simulink model "TVC_model_simulink"  (R2020b)
settings: Solver=VariableStepAuto  StartTime=0.0  StopTime=60  RelTol=1e-3
values from neighbouring files (symbols this model uses):
  C = [1 0 0 0 0 0 ... (first row only)    [TVC_model.m]
  dt = 0.01    [TVC_model.m]
  g = 9.8    [TVC_model.m]
  I = 0.002    [TVC_model.m]
  K = place(A,B,P)    [TVC_model.m]
  L = 0.1    [TVC_model.m]
  m = 1    [TVC_model.m]
undefined symbols (not defined in the file or in its folder): sigbuilder_block
libraries: simulink x1
settings Model: Creator=govindchari  LastModifiedBy=govindchari

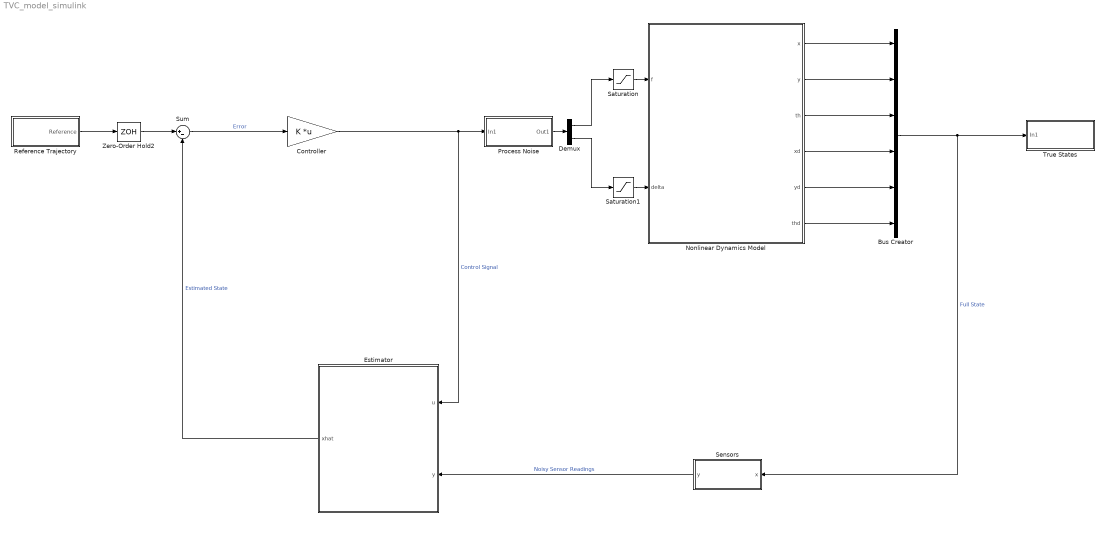
== system TVC_model_simulink ==
  Bus Creator : BusCreator  Inputs=6
  Controller : Gain  Gain=K  Multiplication=Matrix(K*u) (u vector)
  Demux : Demux  Outputs=2
  Estimator : Subsystem
  Nonlinear Dynamics Model : Subsystem
  Process Noise : Subsystem
  Reference Trajectory : Subsystem
  Saturation : Saturate  UpperLimit=m*g  LowerLimit=-m*g
  Saturation1 : Saturate  UpperLimit=0.2  LowerLimit=-0.2
  Sensors : Subsystem
  Sum : Sum  Inputs=|+-
  True States : Subsystem
  Zero-Order Hold2 : ZeroOrderHold  SampleTime=0.01
  wires:
  Nonlinear Dynamics Model/1(x) -> Bus Creator/1
  Nonlinear Dynamics Model/2(y) -> Bus Creator/2
  Nonlinear Dynamics Model/3(th) -> Bus Creator/3
  Nonlinear Dynamics Model/4(xd) -> Bus Creator/4
  Nonlinear Dynamics Model/5(yd) -> Bus Creator/5
  Nonlinear Dynamics Model/6(thd) -> Bus Creator/6
  Bus Creator/1 -> Sensors/1(x), True States/1(In1)  "Full State"
  Demux/1 -> Saturation/1
  Demux/2 -> Saturation1/1
  Sum/1 -> Controller/1  "Error"
  Saturation1/1 -> Nonlinear Dynamics Model/2(delta)
  Saturation/1 -> Nonlinear Dynamics Model/1(f)
  Reference Trajectory/1(Reference) -> Zero-Order Hold2/1
  Zero-Order Hold2/1 -> Sum/1
  Controller/1 -> Estimator/1(u), Process Noise/1(In1)  "Control Signal"
  Process Noise/1(Out1) -> Demux/1
  Sensors/1(y) -> Estimator/2(y)  "Noisy Sensor Readings"
  Estimator/1(xhat) -> Sum/2  "Estimated State"

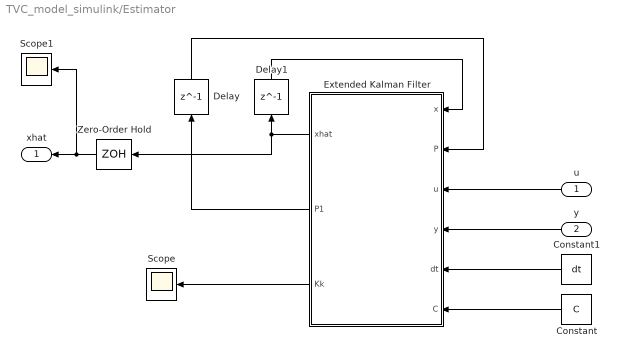
== system TVC_model_simulink/Estimator ==
  u : Inport
  y : Inport  Port=2
  Constant : Constant  Value=C
  Constant1 : Constant  Value=dt
  Delay : Delay  DelayLength=1  InitialCondition=0  SampleTime=dt
  Delay1 : Delay  DelayLength=1  InitialCondition=0  SampleTime=dt
  Extended Kalman Filter : MATLAB Function  TreatAsAtomicUnit=on
  Scope : Scope
  Scope1 : Scope
  Zero-Order Hold : ZeroOrderHold  SampleTime=dt
  xhat : Outport
  wires:
  Delay/1 -> Extended Kalman Filter/2(P)
  Extended Kalman Filter/1(xhat) -> Zero-Order Hold/1, Delay1/1
  Extended Kalman Filter/2(P1) -> Delay/1
  Delay1/1 -> Extended Kalman Filter/1(x)
  y/1 -> Extended Kalman Filter/4(y)
  u/1 -> Extended Kalman Filter/3(u)
  Constant/1 -> Extended Kalman Filter/6(C)
  Constant1/1 -> Extended Kalman Filter/5(dt)
  Zero-Order Hold/1 -> Scope1/1, xhat/1
  Extended Kalman Filter/3(Kk) -> Scope/1

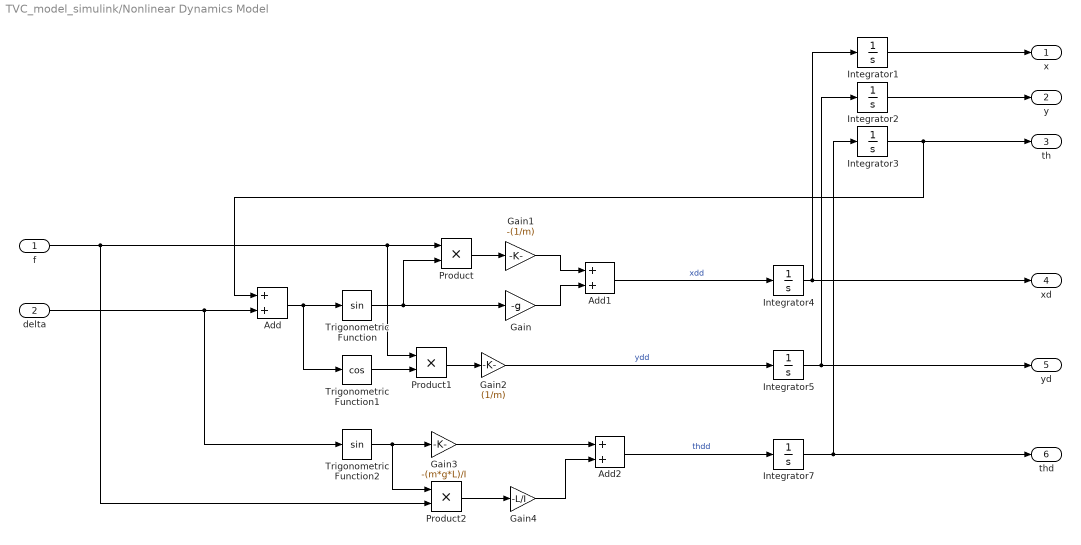
== system TVC_model_simulink/Nonlinear Dynamics Model ==
  f : Inport
  delta : Inport  Port=2
  Add : Sum
  Add1 : Sum
  Add2 : Sum
  Gain : Gain  Gain=-g
  Gain1 : Gain  Gain=-(1/m)
  Gain2 : Gain  Gain=(1/m)
  Gain3 : Gain  Gain=-(m*g*L)/I
  Gain4 : Gain  Gain=-L/I
  Integrator{1..5,7} (6 alike) : Integrator
  Product : Product
  Product1 : Product
  Product2 : Product
  Trigonometric Function : Trigonometry
  Trigonometric Function1 : Trigonometry  Operator=cos
  Trigonometric Function2 : Trigonometry
  x : Outport
  y : Outport  Port=2
  th : Outport  Port=3
  xd : Outport  Port=4
  yd : Outport  Port=5
  thd : Outport  Port=6
  wires:
  Integrator4/1 -> Integrator1/1, xd/1
  Integrator5/1 -> Integrator2/1, yd/1
  Integrator7/1 -> Integrator3/1, thd/1
  Integrator1/1 -> x/1
  Integrator2/1 -> y/1
  Integrator3/1 -> Add/1, th/1
  delta/1 -> Trigonometric Function2/1, Add/2
  Add/1 -> Trigonometric Function1/1, Trigonometric Function/1
  Trigonometric Function/1 -> Product/2, Gain/1
  f/1 -> Product2/2, Product1/1, Product/1
  Product/1 -> Gain1/1
  Gain1/1 -> Add1/1
  Gain/1 -> Add1/2
  Add1/1 -> Integrator4/1  "xdd"
  Trigonometric Function1/1 -> Product1/2
  Product1/1 -> Gain2/1
  Trigonometric Function2/1 -> Product2/1, Gain3/1
  Product2/1 -> Gain4/1
  Gain3/1 -> Add2/1
  Gain4/1 -> Add2/2
  Add2/1 -> Integrator7/1  "thdd"
  Gain2/1 -> Integrator5/1  "ydd"

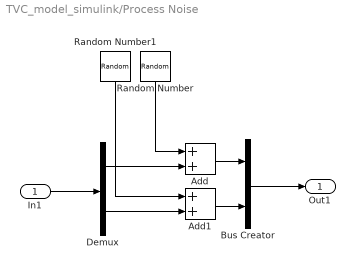
== system TVC_model_simulink/Process Noise ==
  In1 : Inport
  Add : Sum
  Add1 : Sum
  Bus Creator : BusCreator  Inputs=2
  Demux : Demux  Outputs=2
  Random Number : RandomNumber  SampleTime=0.1
  Random Number1 : RandomNumber  Variance=0.0001  SampleTime=0.1
  Out1 : Outport
  wires:
  In1/1 -> Demux/1
  Bus Creator/1 -> Out1/1
  Demux/1 -> Add/2
  Demux/2 -> Add1/2
  Random Number/1 -> Add/1
  Random Number1/1 -> Add1/1
  Add/1 -> Bus Creator/1
  Add1/1 -> Bus Creator/2

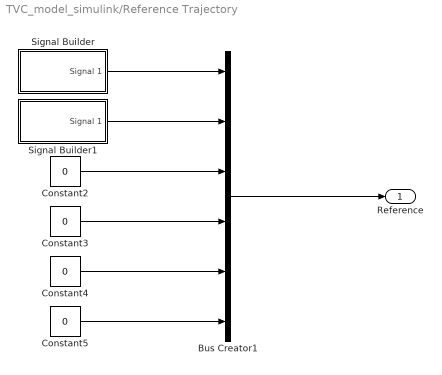
== system TVC_model_simulink/Reference Trajectory ==
  Bus Creator1 : BusCreator  Inputs=6
  Constant{2..5} (4 alike) : Constant  Value=0
  Signal Builder : Subsystem  Tag=STV Subsys  LoadFcn=sigbuilder_block('load');  StartFcn=sigbuilder_block('start');  StopFcn=sigbuilder_block('stop');  ClipboardFcn=sigbuilder_block('clipboard');  mask(Sigbuilder block){tuvar=[0:10]}
      mask help: Simulink:masks:SigbuilderBlock_MD
      mask init:
      | if ~strcmp(get_param(bdroot(gcbh),'SimulationStatus'),'stopped') tuvar = sigbuilder_block('maskInit'); end
      settings: CopyFcn=sigbuilder_block('copy');  DeleteFcn=sigbuilder_block('delete');  ModelCloseFcn=sigbuilder_block('modelClose');  PreSaveFcn=sigbuilder_block('preSave');  PauseFcn=sigbuilder_block('pause');  ContinueFcn=sigbuilder_block('continue');  NameChangeFcn=sigbuilder_block('namechange');  OpenFcn=sigbuilder_block('open',[608 259 753 349 ]);  CloseFcn=sigbuilder_block('close');
      mask Display: plot(0, 0, 100, 100,[2, 2, 32, 32, 2], [68, 8, 8, 68, 68],[32, 2], [38, 38], [32, 19, 2],[53, 60, 44], [32, 17, 17, 2],[16, 16, 31, 31]);txt = getActiveGroup(gcbh);text(2, 100, txt,'verticalAlignment', 'top');
  Signal Builder1 : Subsystem  Tag=STV Subsys  LoadFcn=sigbuilder_block('load');  StartFcn=sigbuilder_block('start');  StopFcn=sigbuilder_block('stop');  ClipboardFcn=sigbuilder_block('clipboard');  mask(Sigbuilder block){tuvar=[0:10]}
      mask help: Simulink:masks:SigbuilderBlock_MD
      mask init:
      | if ~strcmp(get_param(bdroot(gcbh),'SimulationStatus'),'stopped') tuvar = sigbuilder_block('maskInit'); end
      settings: CopyFcn=sigbuilder_block('copy');  DeleteFcn=sigbuilder_block('delete');  ModelCloseFcn=sigbuilder_block('modelClose');  PreSaveFcn=sigbuilder_block('preSave');  PauseFcn=sigbuilder_block('pause');  ContinueFcn=sigbuilder_block('continue');  NameChangeFcn=sigbuilder_block('namechange');  OpenFcn=sigbuilder_block('open',[636 192 753 400 ]);  CloseFcn=sigbuilder_block('close');
      mask Display: plot(0, 0, 100, 100,[2, 2, 32, 32, 2], [68, 8, 8, 68, 68],[32, 2], [38, 38], [32, 19, 2],[53, 60, 44], [32, 17, 17, 2],[16, 16, 31, 31]);txt = getActiveGroup(gcbh);text(2, 100, txt,'verticalAlignment', 'top');
  Reference : Outport
  wires:
  Constant5/1 -> Bus Creator1/6
  Constant3/1 -> Bus Creator1/4
  Constant4/1 -> Bus Creator1/5
  Constant2/1 -> Bus Creator1/3
  Bus Creator1/1 -> Reference/1
  Signal Builder/1(Signal 1) -> Bus Creator1/1
  Signal Builder1/1(Signal 1) -> Bus Creator1/2

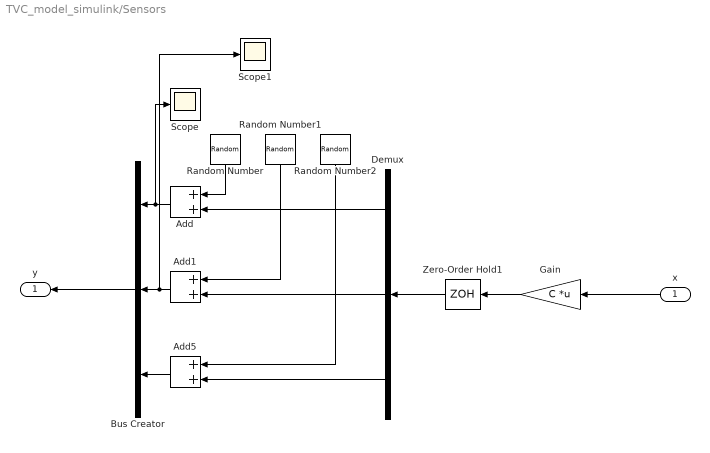
== system TVC_model_simulink/Sensors ==
  x : Inport
  Add : Sum
  Add1 : Sum
  Add5 : Sum
  Bus Creator : BusCreator  Inputs=3
  Demux : Demux  Outputs=3
  Gain : Gain  Gain=C  Multiplication=Matrix(K*u) (u vector)
  Random Number : RandomNumber  SampleTime=dt
  Random Number1 : RandomNumber  Variance=0.01  SampleTime=dt
  Random Number2 : RandomNumber  Variance=0.0001  SampleTime=dt
  Scope : Scope
  Scope1 : Scope
  Zero-Order Hold1 : ZeroOrderHold  SampleTime=0.01
  y : Outport
  wires:
  Bus Creator/1 -> y/1
  Demux/1 -> Add/2
  Demux/2 -> Add1/2
  Add5/1 -> Bus Creator/3
  Add1/1 -> Scope1/1, Bus Creator/2
  Add/1 -> Scope/1, Bus Creator/1
  Random Number/1 -> Add/1
  Random Number1/1 -> Add1/1
  Random Number2/1 -> Add5/1
  Zero-Order Hold1/1 -> Demux/1
  x/1 -> Gain/1
  Gain/1 -> Zero-Order Hold1/1
  Demux/3 -> Add5/2

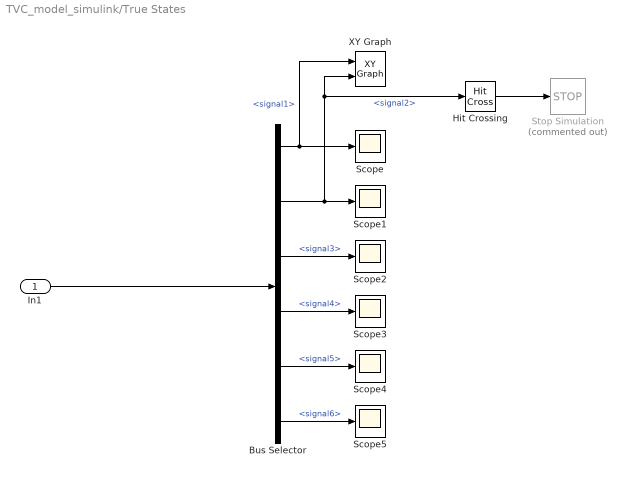
== system TVC_model_simulink/True States ==
  In1 : Inport
  Bus Selector : BusSelector  OutputSignals=signal1,signal2,signal3,signal4,signal5,signal6
  Hit Crossing : HitCross  HitCrossingDirection=falling
  Scope{,1..5} (6 alike) : Scope
  Stop Simulation : Stop  Commented=on
  XY Graph : simulink/Sinks/XY Graph  xmin=-10  xmax=70  ymin=-10  ymax=30  st=-1
  wires:
  In1/1 -> Bus Selector/1
  Bus Selector/2 -> Hit Crossing/1, XY Graph/2, Scope1/1  "<signal2>"
  Hit Crossing/1 -> Stop Simulation/1
  Bus Selector/1 -> XY Graph/1, Scope/1  "<signal1>"
  Bus Selector/5 -> Scope4/1  "<signal5>"
  Bus Selector/4 -> Scope3/1  "<signal4>"
  Bus Selector/6 -> Scope5/1  "<signal6>"
  Bus Selector/3 -> Scope2/1  "<signal3>"

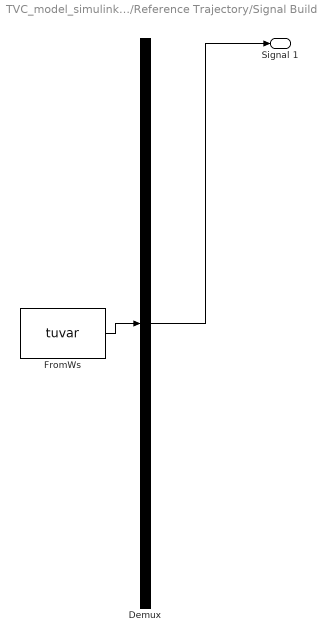
== system TVC_model_simulink/Reference Trajectory/Signal Builder ==
  Demux : Demux  Tag=STV Demux  Outputs=1
      settings: DisplayOption=none
  FromWs : FromWorkspace  Tag=STV FromWs  VariableName=tuvar
      SigBuilderData=|
      | common.afterFinalStr = 'Extrapolate'
      | common.sampleTime = 0
      | dataSet.timeRange = [0 55]
      | dataSet.name = 'Group 1'
      | sbobj.Groups.Name = 'Group 1'
      | sbobj.Groups.Signals.Name = 'Signal 1'
      | sbobj.Groups.Signals.XData = [0 15 40 55]
      | sbobj.Groups.Signals.YData = [0 0 50 50]
      | sbobj.Groups.TimeRange = [0 55]
  Signal 1 : Outport  Tag=STV Outport
  wires:
  Demux/1 -> Signal 1/1
  FromWs/1 -> Demux/1

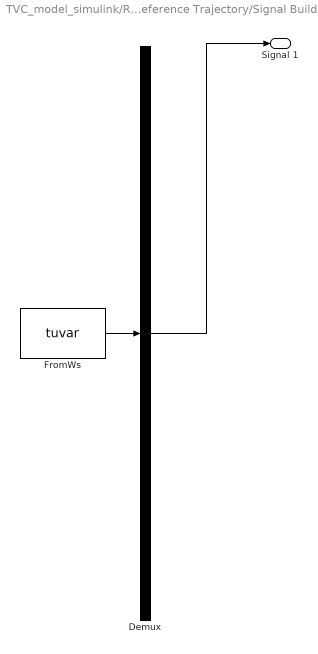
== system TVC_model_simulink/Reference Trajectory/Signal Builder1 ==
  Demux : Demux  Tag=STV Demux  Outputs=1
      settings: DisplayOption=none
  FromWs : FromWorkspace  Tag=STV FromWs  VariableName=tuvar
      SigBuilderData=|
      | common.afterFinalStr = 'Extrapolate'
      | common.sampleTime = 0
      | dataSet.timeRange = [0 55]
      | dataSet.name = 'Group 1'
      | sbobj.Groups.Name = 'Group 1'
      | sbobj.Groups.Signals.Name = 'Signal 1'
      | sbobj.Groups.Signals.XData = [0 15 40 55 55]
      | sbobj.Groups.Signals.YData = [0 20 20 0 0]
      | sbobj.Groups.TimeRange = [0 55]
  Signal 1 : Outport  Tag=STV Outport
  wires:
  Demux/1 -> Signal 1/1
  FromWs/1 -> Demux/1

== matlab function TVC_model_simulink/Estimator/Extended Kalman Filter ==
  data: x input; P input; u input; y input; xhat output; P1 output; dt input; C input; Kk output
function [xhat,P1,Kk] = EKF(x,P,u,y,dt,C)
    f=u(1);
    delta=u(2);
    m=1;
    g=9.8;
    L=0.2;
    I=0.002;

    %Process Noise Covariance
    Q=[0 0 0 0 0 0;
       0 0 0 0 0 0;
       0 0 0 0 0 0;
       0 0 0 0.0096 0 0.4802;
       0 0 0 0 1 0;
       0 0 0 0.4802 0 24.0100];
    
    %Sensor Noise Covariance
    R=diag([0.9 0.01 0.005]);
    
    if size(x)==1
        x0=zeros(6,1);
        P0=eye(6);
    else
        x0=x;
        P0=P;
    end
    
    %State Transition Matrix (Jacobian of Nonlinear State Transition)
    F=[1 0 0 dt 0 0;
       0 1 0 0 dt 0;
       0 0 1 0 0 dt;
       0 0 -dt*cos(delta+x0(3))*(g+f/m) 1 0 0;
       0 0 -dt*sin(delta+x0(3))*(f/m) 0 1 0;
       0 0 0 0 0 1];
   
    %Nonlinear State Propagation to get predicted xhat
    x1_p=[x0(4)*dt+x0(1);
          x0(5)*dt+x0(2);
          x0(6)*dt+x0(3);
          -dt*sin(delta+x0(3))*(g+f/m)+x0(4);
          dt*cos(delta+x0(3))*(f/m)+x0(5);
          -dt*sin(delta)*(m*g*L/I+f*L/I)+x0(6)];
      
    %Linearized Covariance Propagation to get predicted P
    P1_p=F*P0*F.'+Q;
    
    %Total Error
    S=C*P1_p*C.'+R;
    
    %Kalman Gain
    Kk=P1_p*C.'*S^-1;
    
    %Outputs
    xhat=x1_p+Kk*(y-C*x1_p);
    P1=(eye(6)-Kk*C)*P1_p;
